simulink model "driveline_springdamper_flex"  (R2016b)
settings: Solver=ode4  StartTime=0.0  StopTime=10.0  FixedStep=0.01  RelTol=1e-3
libraries: fl_lib x4, nesl_utility x3, sdl_lib x1
settings Model: TunableVars=A  TunableVarsStorageClass=Auto  Creator=jgillis  LastModifiedBy=jgillis
settings OptimizationCC: EnableMemcpy=off
settings RTWCC: RTWVerbose=off
settings SimscapeCC: SimscapeLogType=all  SimscapeLogLimitData=off  SimscapeLogDataHistory=1000

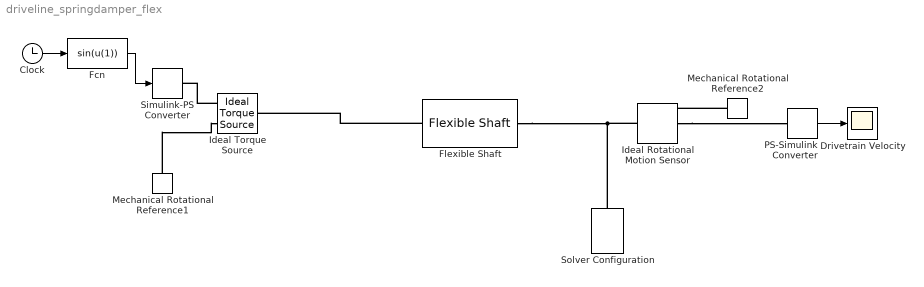
== system driveline_springdamper_flex ==
  Clock : Clock
  Drivetrain Velocity : Scope
  Fcn : Fcn  Expr=sin(u(1))
  Flexible Shaft : sdl_lib/Couplings & Drives/Flexible Shaft  parameterization=1  shaft_stiffness=1 N*m/rad  shaft_inertia=0.02 kg*m^2  shaft_construction=1  length=1 m  diameter_outer=0.075 m  diameter_inner=0.05 m  density=7.8e+3 kg/m^3  shear_modulus=7.93e+10 Pa  damping_ratio=0.01  n_segments=1  mu_visc=[ 0 0 ] N*m/(rad/s)  initial_deflection=0 rad  initial_velocity=0 rpm
  Ideal Rotational Motion Sensor : fl_lib/Mechanical/Mechanical Sensors/Ideal Rotational Motion Sensor  offset=0 rad
  Ideal Torque Source : fl_lib/Mechanical/Mechanical Sources/Ideal Torque Source
  Mechanical Rotational Reference1 : fl_lib/Mechanical/Rotational Elements/Mechanical Rotational Reference
  Mechanical Rotational Reference2 : fl_lib/Mechanical/Rotational Elements/Mechanical Rotational Reference
  PS-Simulink Converter : nesl_utility/PS-Simulink Converter  PhysicalDomain=network_engine_domain  SubClassName=ps_output  LeftPortType=input  RightPortType=output  PseudoPeriodic=off  Frequencies=[]  Unit=1  AffineConversion=off
  Simulink-PS Converter : nesl_utility/Simulink-PS Converter  PhysicalDomain=network_engine_domain  SubClassName=ps_input  LeftPortType=input  RightPortType=output  PseudoPeriodic=off  Frequencies=[]  NoiseDistribution=none  NoiseParameters=[]  Unit=1  AffineConversion=off  InputFiltering=off  SimscapeFilterOrder=1  InputFilterTimeConstant=0.001  UdotUserProvided=1
  Solver Configuration : nesl_utility/Solver Configuration  PhysicalDomain=network_engine_domain  SubClassName=solver  LeftPortType=input  RightPortType=generic  Accelerate=off  Tones=[]  Harmonics=[]  SimulateNoise=off  Profile=off  UseLocalSampling=off  EnableSwitchedLinearOptims=on  FrequencyDomain=off  UseCCode=off  RelTol=0.001  AbsTol=1e-06  MinStep=1e-09  ToWorkspace=off  RevertToSquareIcSolve=off  NumHomotopyIterations=100  PhasorMode=off  PhasorModeNumHarmonics=1  OverrideAbsTol=off  DoDC=off  ResidualTolerance=1e-9  UseLocalSolver=on  LocalSolverChoice=NE_BACKWARD_EULER_ADVANCER  LocalSolverSampleTime=0.01  DoFixedCost=on  MaxNonlinIter=10  MaxModeIter=2  LinearAlgebra=Sparse  DelaysMemoryBudget=1024  AutomaticFiltering=on  FilteringTimeConstant=0.001
  wires:
  Clock/1 -> Fcn/1
  Fcn/1 -> Simulink-PS Converter/1
  PS-Simulink Converter/1 -> Drivetrain Velocity/1
  connections:
  Ideal Torque Source/RConn1 -- Simulink-PS Converter/RConn1
  Flexible Shaft/LConn1 -- Ideal Torque Source/LConn1
  Ideal Rotational Motion Sensor/LConn1 -- Flexible Shaft/RConn1 -- Solver Configuration/RConn1
  Ideal Rotational Motion Sensor/RConn2 -- PS-Simulink Converter/LConn1
  Mechanical Rotational Reference1/LConn1 -- Ideal Torque Source/RConn2
  Mechanical Rotational Reference2/LConn1 -- Ideal Rotational Motion Sensor/RConn1
